simulink library "mpcgpkf_altitudeOptimization"  (R2020a)
settings: Solver=VariableStepAuto  StartTime=0.0  StopTime=10.0  RelTol=1e-3
values from neighbouring files (symbols this model uses):
  Amat = block.DialogPrm(1).Data    [altOptMPC_level2SFunc.m]    (also in kfgpPrediction_init.m = kron(eye(nAlt),F))
  Hmat = block.DialogPrm(3).Data    [altOptMPC_level2SFunc.m]    (also in kfgpPrediction_init.m = kron(eye(nAlt),H))
  Ks = block.DialogPrm(5).Data    [altOptMPC_level2SFunc.m]    (also in kfgpPrediction_init.m = Ks + triu(Ks,1)'; kfgp_init.m = spatialCovariance(xMeasure(:),xMeasure(:),covAmp,spatialScal)
  Ks12 = block.DialogPrm(6).Data    [altOptMPC_level2SFunc.m]    (also in kfgpPrediction_init.m = sqrtm(Ks); kfgp_init.m = sqrtm(Ks))
  Qmat = block.DialogPrm(2).Data    [altOptMPC_level2SFunc.m]    (also in kfgpPrediction_init.m = kron(eye(nAlt),Q))
  Rmat = block.DialogPrm(4).Data    [altOptMPC_level2SFunc.m]    (also in kfgpPrediction_init.m = R)
libraries: simulink x1
settings Model: Creator=Ayaz  LastModifiedBy=Ayaz

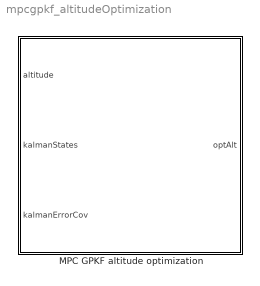
== system mpcgpkf_altitudeOptimization ==
  MPC GPKF altitude optimization : Subsystem  mask{timeScale=22*60, spatialScale=220, covAmp=1, xMeasure=100:100:1000, noiseVar=0.01, hTau='exponential', powerLawParams=[3.77 0.14], mpcgpkfTimeStep=10, nPred=6, zMax=1000, zMin=100, zStepMax=100, tradeoffCons=5}
      mask prompts: timeScale "Temporal length scale [s]"; spatialScale "Altitude lenght scale [m]"; covAmp "Altitude covariance amplitude [-]"; xMeasure "Discreted altitudes measurement space [m]"; noiseVar "Noise variance [m^2/s^2]"; hTau "Temporal kernel"; powerLawParams "Power law parameters, mZ = a*z^b"; mpcgpkfTimeStep "Time step [s]"; nPred "Prediction horizon"; zMax "Maximum altitude"; zMin "Mimimum altitude"; zStepMax "Max altitude change"; tradeoffCons "Tradeoff constant"
      mask init:
      | [Amat,Qmat,Hmat,Rmat,Ks,Ks12,s0,sigma0] = kfgp_init(xMeasure,covAmp,...
      |     spatialScale,noiseVar,hTau,mpcgpkfTimeStep,timeScale);
      mask DialogControl ParameterGroupVar Prompt: GPKF parameters
      mask DialogControl Container3 Prompt: MPC parameters

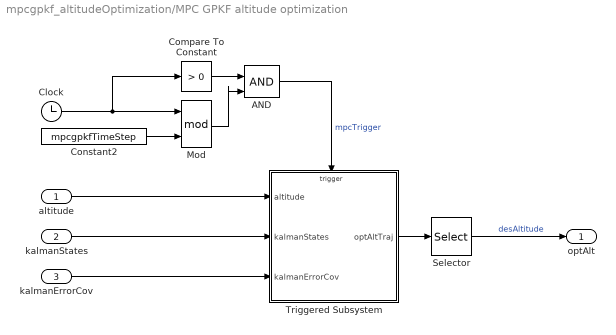
== system mpcgpkf_altitudeOptimization/MPC GPKF altitude optimization ==
  altitude : Inport
  kalmanStates : Inport  Port=2
  kalmanErrorCov : Inport  Port=3
  AND : Logic  IconShape=distinctive  AllPortsSameDT=off  OutDataTypeStr=boolean
  Clock : Clock
  Compare To Constant : simulink/Logic and Bit Operations/Compare To Constant  relop=>  const=0  OutDataTypeStr=boolean
  Constant2 : Constant  Value=mpcgpkfTimeStep  VectorParams1D=off
  Mod : Math  Operator=mod  SaturateOnIntegerOverflow=on
  Selector : Selector  InputPortWidth=nPred  IndexOptions=Index vector (dialog)  Indices=1  OutputSizes=1
  Triggered Subsystem : Subsystem  TreatAsAtomicUnit=on
  optAlt : Outport
  wires:
  altitude/1 -> Triggered Subsystem/1(altitude)
  kalmanStates/1 -> Triggered Subsystem/2(kalmanStates)
  kalmanErrorCov/1 -> Triggered Subsystem/3(kalmanErrorCov)
  Triggered Subsystem/1(optAltTraj) -> Selector/1
  Mod/1 -> AND/2
  Constant2/1 -> Mod/2
  Clock/1 -> Compare To Constant/1, Mod/1
  Compare To Constant/1 -> AND/1
  AND/1 -> Triggered Subsystem/Trigger  "mpcTrigger"
  Selector/1 -> optAlt/1  "desAltitude"

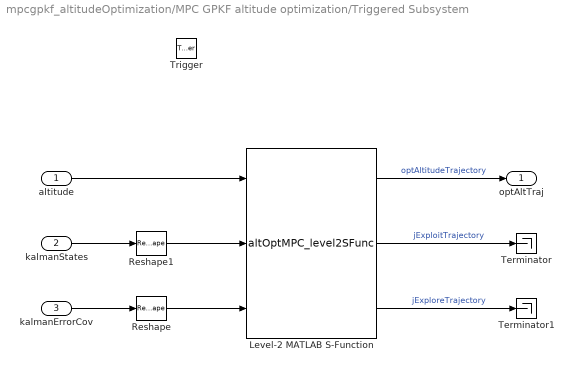
== system mpcgpkf_altitudeOptimization/MPC GPKF altitude optimization/Triggered Subsystem ==
  altitude : Inport
  kalmanStates : Inport  Port=2
  kalmanErrorCov : Inport  Port=3
  Trigger : TriggerPort  VariantControl=Variant
  Level-2 MATLAB S-Function : M-S-Function  FunctionName=altOptMPC_level2SFunc  Parameters=Amat,Qmat,Hmat,Rmat,Ks,Ks12,covAmp,spatialScale,xMeasure,powerLawParams,nPred,zMin,zMax,zStepMax,tradeoffCons
  Reshape : Reshape
  Reshape1 : Reshape
  Terminator : Terminator
  Terminator1 : Terminator
  optAltTraj : Outport
  wires:
  kalmanStates/1 -> Reshape1/1
  kalmanErrorCov/1 -> Reshape/1
  Level-2 MATLAB S-Function/1 -> optAltTraj/1  "optAltitudeTrajectory"
  altitude/1 -> Level-2 MATLAB S-Function/1
  Reshape1/1 -> Level-2 MATLAB S-Function/2
  Reshape/1 -> Level-2 MATLAB S-Function/3
  Level-2 MATLAB S-Function/2 -> Terminator/1  "jExploitTrajectory"
  Level-2 MATLAB S-Function/3 -> Terminator1/1  "jExploreTrajectory"
